simulink model "Copy_of_LoopShapingTOT"  (R2019b)
settings: Solver=ode45  StartTime=0.0  StopTime=20  RelTol=1e-3  EnableMultiTasking=on
values from neighbouring files (symbols this model uses):
  m = 0.5    [LCS_freq.m]    (also in LoopShaping_TP.m = 2)
libraries: simulink x1
settings Model: Creator=Kathleeen  LastModifiedBy=Ivan
settings DataIOCC: LimitDataPoints=on  SaveFormat=Array  ReturnWorkspaceOutputs=off
settings OptimizationCC: LifeSpan=inf
settings DebuggingCC: UnderspecifiedInitializationDetection=Classic  MergeDetectMultiDrivingBlocksExec=none  StateNameClashWarn=warning  SFUnexpectedBacktrackingDiag=warning  SFNoUnconditionalDefaultTransitionDiag=warning  SFExecutionAtInitializationDiag=none  ArithmeticOperatorsInVariantConditions=warning
settings HardwareCC: ProdBitPerPointer=32  ProdBitPerSizeT=32  ProdBitPerPtrDiffT=32  ProdLargestAtomicFloat=None  ProdIntDivRoundTo=Undefined  ProdEndianess=Unspecified  ProdWordSize=32  ProdHWDeviceType=32-bit Generic
settings ModelReferenceCC: PropagateSignalLabelsOutOfModel=off
settings SFSimCC: SimUseLocalCustomCode=off  CustomCodeUndefinedFunction=UseInterfaceOnly
settings RTWCC: RTWUseLocalCustomCode=off
settings CodeAppCC: StateflowObjectComments=on
settings GRTTargetCC: TargetLangStandard=C89/C90 (ANSI)  GeneratePreprocessorConditionals=Disable all
settings ConfigComp: CovMetricSettings=dw  CovHtmlReporting=on  CovSaveCumulativeToWorkspaceVar=on  CovSaveSingleToWorkspaceVar=on  CovExternalEMLEnable=off

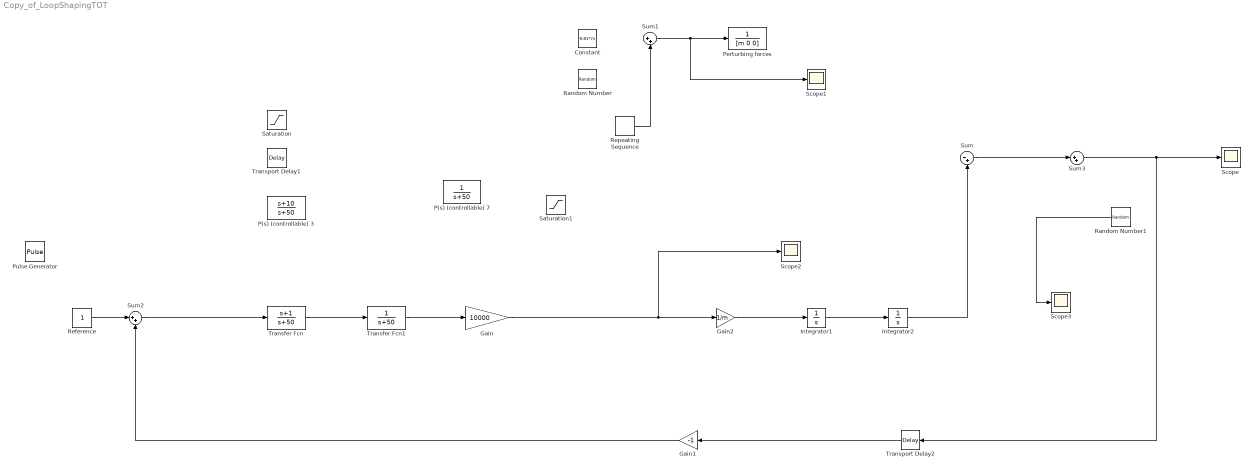
== system Copy_of_LoopShapingTOT ==
  Constant : Constant  Value=9.81*m
  Gain : Gain  Gain=10000
  Gain1 : Gain  Gain=-1
  Gain2 : Gain  Gain=1/m
  Integrator1 : Integrator
  Integrator2 : Integrator
  P(s) (controllable) 3 : TransferFcn  Numerator=[1 10]  Denominator=[1 50]
  P(s) (controllable) 7 : TransferFcn  Denominator=[1 50]
  "Perturbing forces " : TransferFcn  Denominator=[m 0 0]
  Pulse Generator : DiscretePulseGenerator  PulseType=Time based  Amplitude=0.5  Period=5  PulseWidth=50
  Random Number : RandomNumber  Seed=3  SampleTime=0.01
  Random Number1 : RandomNumber  Variance=0.0001  Seed=3  SampleTime=0.01
  "Reference " : Constant
  Repeating Sequence : simulink/Sources/Repeating Sequence  rep_seq_t=[0 2]  rep_seq_y=[0 1]
  Saturation : Saturate
  Saturation1 : Saturate  UpperLimit=10  LowerLimit=-10
  Scope{,1..3} (4 alike) : Scope
  Sum : Sum  Inputs=|-+
  Sum1 : Sum  Inputs=|++
  Sum2 : Sum  Inputs=|++
  Sum3 : Sum  Inputs=|++
  Transfer Fcn : TransferFcn  Numerator=[1 1]  Denominator=[1 50]
  Transfer Fcn1 : TransferFcn  Denominator=[1 50]
  Transport Delay1 : TransportDelay
  Transport Delay2 : TransportDelay  DelayTime=0.05
  wires:
  Integrator2/1 -> Sum/2
  "Reference "/1 -> Sum2/1
  Integrator1/1 -> Integrator2/1
  Gain2/1 -> Integrator1/1
  Random Number1/1 -> Scope3/1
  Sum1/1 -> Scope1/1, "Perturbing forces "/1
  Gain1/1 -> Sum2/2
  Sum/1 -> Sum3/1
  Transfer Fcn1/1 -> Gain/1
  Transfer Fcn/1 -> Transfer Fcn1/1
  Repeating Sequence/1 -> Sum1/2
  Sum3/1 -> Transport Delay2/1, Scope/1
  Gain/1 -> Gain2/1, Scope2/1
  Sum2/1 -> Transfer Fcn/1
  Transport Delay2/1 -> Gain1/1
